simulink model "nms_model_nonlin"  (R2020a)
settings: Solver=VariableStepAuto  StartTime=0.0  StopTime=7  FixedStep=0.0001  MaxStep=.01  RelTol=1e-4  AbsTol=1e-6
values from neighbouring files (symbols this model uses):
  animFrameRate = 10    [runmodel.m]
  dt_visual = -1    [NMScontrol.m]    (also in runmodel.m = 0.001)
  g = params.g    [NMPCcostFunction.m]    (also in dynamicsNMPC.m = 9.81)
  m = parametersOpt(1)    [CGBgreybox.m]    (also in NMPCcostFunction.m = params.m)
  params = setupParamsStruct(parametersOpt, dt, controlParams)    [CGBcontrol.m]    (also in CGBgreybox.m = setupParamsStruct(parametersOpt); computationTime.m = setupParamsStruct(ParametersOpt, Qy, yref, dt))
undefined symbols (not defined in the file or in its folder): footMass, hatLeftHipToCenterDistWidth, hatMass, initialTargetAngle, legMass, LongDelay, LongLoopDelay, LPreStimBFSHinit, LPreStimGASinit, LPreStimGLUinit, LPreStimHABinit, LPreStimHADinit, LPreStimHAMinit, LPreStimHFLinit, LPreStimRFinit, LPreStimSOLinit, LPreStimTAinit, LPreStimVASinit, LTargetAngleInit, LTargetAngleRInit, MidDelay, RPreStimBFSHinit, RPreStimGASinit, RPreStimGLUinit, RPreStimHABinit, RPreStimHADinit, RPreStimHAMinit, RPreStimHFLinit, RPreStimRFinit, RPreStimSOLinit, RPreStimTAinit, RPreStimVASinit, RTargetAngleInit, RTargetAngleRInit, shankLength, shankMass, ShortDelay, termination_height, thetaHATref, thighLength, thighMass, totalMass, X, Y, Z
libraries: NeuroMuscularLibrary x113, nesl_utility x30, sm_lib x24, simulink x3
(part 5 of 5)

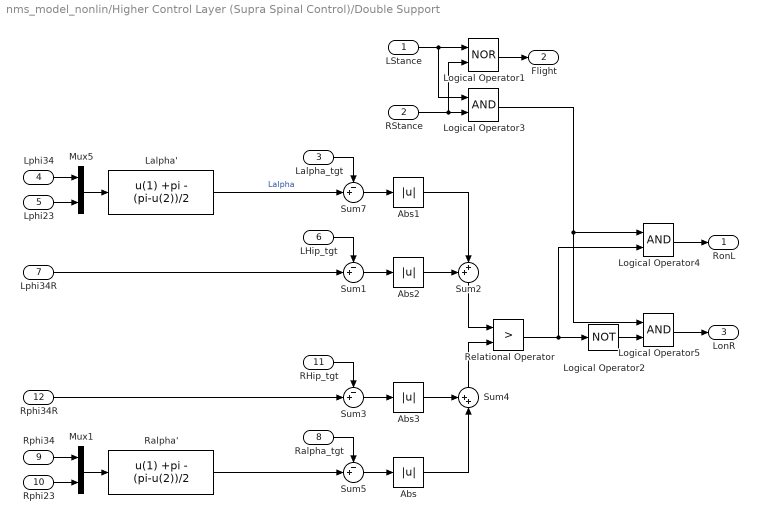
== system nms_model_nonlin/Higher Control Layer (Supra Spinal Control)/Double Support ==
  LStance : Inport
  RStance : Inport  Port=2
  Lalpha_tgt : Inport  Port=3
  Lphi34 : Inport  Port=4
  Lphi23 : Inport  Port=5
  LHip_tgt : Inport  Port=6
  Lphi34R : Inport  Port=7
  Ralpha_tgt : Inport  Port=8
  Rphi34 : Inport  Port=9
  Rphi23 : Inport  Port=10
  RHip_tgt : Inport  Port=11
  Rphi34R : Inport  Port=12
  Abs{,1..3} (4 alike) : Abs  ZeroCross=off
  Lalpha' : Fcn  Expr=u(1) +pi - (pi-u(2))/2
  Logical Operator1 : Logic  Operator=NOR  AllPortsSameDT=off  OutDataTypeStr=boolean
  Logical Operator2 : Logic  Operator=NOT  AllPortsSameDT=off
  Logical Operator3 : Logic  AllPortsSameDT=off
  Logical Operator4 : Logic  AllPortsSameDT=off
  Logical Operator5 : Logic  AllPortsSameDT=off
  Mux1 : Mux  Inputs=2
  Mux5 : Mux  Inputs=2
  Ralpha' : Fcn  Expr=u(1) +pi - (pi-u(2))/2
  Relational Operator : RelationalOperator  Operator=>  ZeroCross=off  RndMeth=Nearest
  Sum{1,3,5,7} (4 alike) : Sum  Inputs=-+|
  Sum2 : Sum  Inputs=++|
  Sum4 : Sum  Inputs=++|
  RonL : Outport
  Flight : Outport  Port=2
  LonR : Outport  Port=3
  wires:
  Lalpha'/1 -> Sum7/2  "Lalpha"
  Mux5/1 -> Lalpha'/1
  Ralpha'/1 -> Sum5/2
  Mux1/1 -> Ralpha'/1
  Sum5/1 -> Abs/1
  Sum7/1 -> Abs1/1
  LStance/1 -> Logical Operator3/1, Logical Operator1/1
  RStance/1 -> Logical Operator3/2, Logical Operator1/2
  Lalpha_tgt/1 -> Sum7/1
  Lphi34/1 -> Mux5/1
  Lphi23/1 -> Mux5/2
  Ralpha_tgt/1 -> Sum5/1
  Rphi34/1 -> Mux1/1
  Rphi23/1 -> Mux1/2
  Logical Operator1/1 -> Flight/1
  LHip_tgt/1 -> Sum1/1
  Lphi34R/1 -> Sum1/2
  Sum1/1 -> Abs2/1
  Abs2/1 -> Sum2/1
  Abs1/1 -> Sum2/2
  Sum2/1 -> Relational Operator/1
  RHip_tgt/1 -> Sum3/1
  Rphi34R/1 -> Sum3/2
  Sum3/1 -> Abs3/1
  Abs/1 -> Sum4/2
  Abs3/1 -> Sum4/1
  Sum4/1 -> Relational Operator/2
  Logical Operator4/1 -> RonL/1
  Logical Operator2/1 -> Logical Operator5/2
  Logical Operator5/1 -> LonR/1
  Relational Operator/1 -> Logical Operator2/1, Logical Operator4/2
  Logical Operator3/1 -> Logical Operator5/1, Logical Operator4/1

== system nms_model_nonlin/Body Mechanics Layer/state sensor/If Action Subsystem ==
  In1 : Inport
  Action Port : ActionPort  ActionPortLabel=if(u2==3|u2==4)
  Out1 : Outport
  wires:
  In1/1 -> Out1/1

== system nms_model_nonlin/Body Mechanics Layer/state sensor/If Action Subsystem1 ==
  In1 : Inport
  Action Port : ActionPort  ActionPortLabel=else
  Out1 : Outport
  wires:
  In1/1 -> Out1/1

== matlab function nms_model_nonlin/Body Mechanics Layer/MPC ==
  data: x input; y output; params parameter
function y = fcn(x, params)
    coder.extrinsic('NMPC_mex'); 
    counter = x(7);
    if x(6) == 0
        counter = 0;
    elseif x(6) == 1
        counter = counter + 1;
    end
    kimp = 49-counter;
    if x(6) == 1
        dt = params.dt;
%         timp = heelstrike(x(1:4),params); % Find when heelstrike occurs
%         kimp = round(timp/dt);
        if kimp > 0
            % Prosthetic swing
            uoptvector = NMPC_mex(x(1:4), kimp, params);
            uopt = uoptvector(1);
        else
            uopt = 0;
        end
    else
        uopt = 0;
        kimp = 0;
    end
    y = zeros(2,1);
    y(1) = uopt;
    y(2) = counter;
end
